simulink model "Exercitiul4_1"  (R2016a)
settings: Solver=VariableStepDiscrete  StartTime=0.0  StopTime=100  RelTol=1e-3
undefined symbols (not defined in the file): exprnd, m
settings Model: Creator=Cristina  LastModifiedBy=Cristina

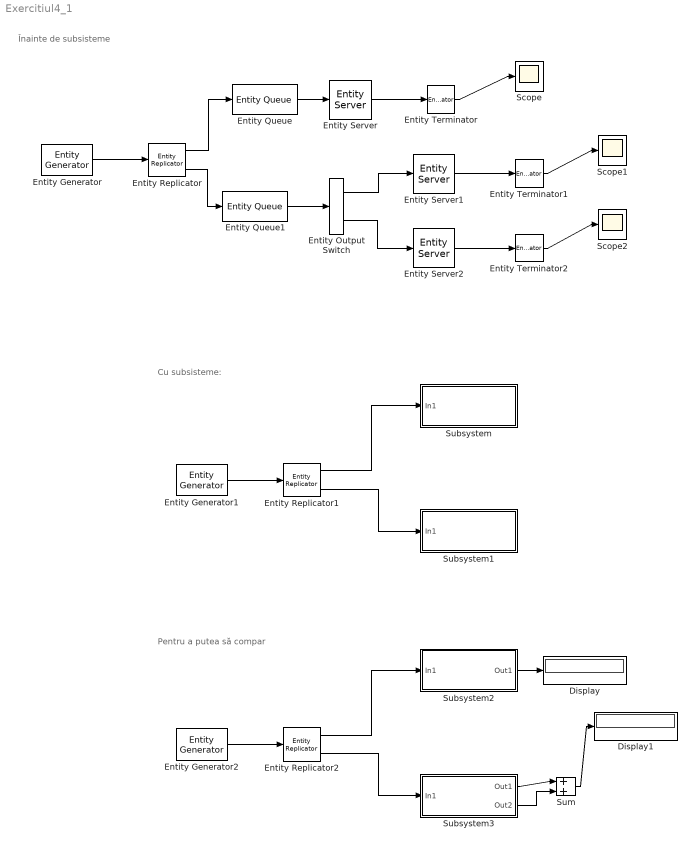
== system Exercitiul4_1 ==
  note: Cu subsisteme:
  note: Înainte de subsisteme
  note: Pentru a putea să compar
  Display : Display
  Display1 : Display
  Entity Output Switch : EntityOutputSwitch  InputPortMessageModes=m  OutputPortMessageModes=m,m  SwitchAttributeName=Attribute1
  Entity Generator : EntityGenerator  OutputPortMessageModes=m  TimeSource=MATLAB action  IntergenerationTimeAction=dt = exprnd(0.5);  AttributeName=ServiceTime  AttributeInitialValue=exprnd(1)  EntityType=Structured  EntityTypeName=Entity
  Entity Generator1 : EntityGenerator  OutputPortMessageModes=m  TimeSource=MATLAB action  IntergenerationTimeAction=dt = exprnd(0.5);  AttributeName=ServiceTime  AttributeInitialValue=exprnd(1)  EntityType=Structured  EntityTypeName=Entity
  Entity Generator2 : EntityGenerator  OutputPortMessageModes=m  TimeSource=MATLAB action  IntergenerationTimeAction=dt = exprnd(0.5);  AttributeName=ServiceTime  AttributeInitialValue=exprnd(1)  EntityType=Structured  EntityTypeName=Entity
  Entity Queue : EntityQueue  InputPortMessageModes=m  OutputPortMessageModes=m
      settings: OutputPortMap=o5
  Entity Queue1 : EntityQueue  InputPortMessageModes=m  OutputPortMessageModes=m
      settings: OutputPortMap=o5
  Entity Replicator : EntityReplicator  InputPortMessageModes=m  OutputPortMessageModes=m,m
  Entity Replicator1 : EntityReplicator  InputPortMessageModes=m  OutputPortMessageModes=m,m
  Entity Replicator2 : EntityReplicator  InputPortMessageModes=m  OutputPortMessageModes=m,m
  Entity Server : EntityServer  InputPortMessageModes=m  OutputPortMessageModes=m  Capacity=2  ServiceTimeSource=Attribute
  Entity Server1 : EntityServer  InputPortMessageModes=m  OutputPortMessageModes=m  Capacity=1  ServiceTimeSource=Attribute
  Entity Server2 : EntityServer  InputPortMessageModes=m  OutputPortMessageModes=m  Capacity=1  ServiceTimeSource=Attribute
  Entity Terminator : EntityTerminator  InputPortMessageModes=m  NumberEntitiesArrived=on
      settings: OutputPortMap=o0
  Entity Terminator1 : EntityTerminator  InputPortMessageModes=m  NumberEntitiesArrived=on
      settings: OutputPortMap=o0
  Entity Terminator2 : EntityTerminator  InputPortMessageModes=m  NumberEntitiesArrived=on
      settings: OutputPortMap=o0
  Scope : Scope
  Scope1 : Scope
  Scope2 : Scope
  Subsystem : Subsystem
  Subsystem1 : Subsystem
  Subsystem2 : Subsystem
  Subsystem3 : Subsystem
  Sum : Sum  Inputs=|++
  wires:
  Entity Replicator/1 -> Entity Queue/1
  Entity Generator/1 -> Entity Replicator/1
  Entity Replicator/2 -> Entity Queue1/1
  Entity Queue/1 -> Entity Server/1
  Entity Queue1/1 -> Entity Output Switch/1
  Entity Output Switch/1 -> Entity Server1/1
  Entity Output Switch/2 -> Entity Server2/1
  Entity Server/1 -> Entity Terminator/1
  Entity Server1/1 -> Entity Terminator1/1
  Entity Server2/1 -> Entity Terminator2/1
  Entity Terminator/1 -> Scope/1
  Entity Terminator1/1 -> Scope1/1
  Entity Terminator2/1 -> Scope2/1
  Entity Generator1/1 -> Entity Replicator1/1
  Entity Replicator1/2 -> Subsystem1/1(In1)
  Entity Replicator1/1 -> Subsystem/1(In1)
  Entity Generator2/1 -> Entity Replicator2/1
  Entity Replicator2/2 -> Subsystem3/1(In1)
  Entity Replicator2/1 -> Subsystem2/1(In1)
  Subsystem2/1(Out1) -> Display/1
  Subsystem3/1(Out1) -> Sum/1
  Subsystem3/2(Out2) -> Sum/2
  Sum/1 -> Display1/1

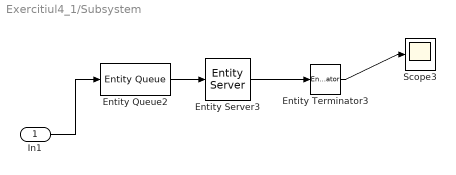
== system Exercitiul4_1/Subsystem ==
  In1 : Inport
  Entity Queue2 : EntityQueue  InputPortMessageModes=m  OutputPortMessageModes=m
      settings: OutputPortMap=o5
  Entity Server3 : EntityServer  InputPortMessageModes=m  OutputPortMessageModes=m  Capacity=2  ServiceTimeSource=Attribute
  Entity Terminator3 : EntityTerminator  InputPortMessageModes=m  NumberEntitiesArrived=on
      settings: OutputPortMap=o0
  Scope3 : Scope
  wires:
  In1/1 -> Entity Queue2/1
  Entity Queue2/1 -> Entity Server3/1
  Entity Server3/1 -> Entity Terminator3/1
  Entity Terminator3/1 -> Scope3/1

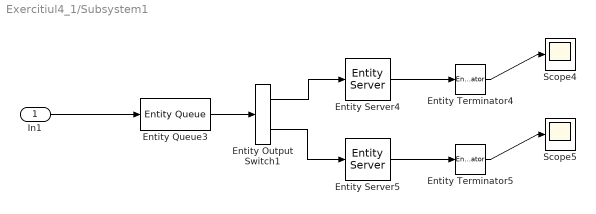
== system Exercitiul4_1/Subsystem1 ==
  In1 : Inport
  Entity Output Switch1 : EntityOutputSwitch  InputPortMessageModes=m  OutputPortMessageModes=m,m  SwitchAttributeName=Attribute1
  Entity Queue3 : EntityQueue  InputPortMessageModes=m  OutputPortMessageModes=m
      settings: OutputPortMap=o5
  Entity Server4 : EntityServer  InputPortMessageModes=m  OutputPortMessageModes=m  Capacity=1  ServiceTimeSource=Attribute
  Entity Server5 : EntityServer  InputPortMessageModes=m  OutputPortMessageModes=m  Capacity=1  ServiceTimeSource=Attribute
  Entity Terminator4 : EntityTerminator  InputPortMessageModes=m  NumberEntitiesArrived=on
      settings: OutputPortMap=o0
  Entity Terminator5 : EntityTerminator  InputPortMessageModes=m  NumberEntitiesArrived=on
      settings: OutputPortMap=o0
  Scope4 : Scope
  Scope5 : Scope
  wires:
  Entity Queue3/1 -> Entity Output Switch1/1
  Entity Output Switch1/1 -> Entity Server4/1
  Entity Output Switch1/2 -> Entity Server5/1
  Entity Server4/1 -> Entity Terminator4/1
  Entity Server5/1 -> Entity Terminator5/1
  Entity Terminator4/1 -> Scope4/1
  Entity Terminator5/1 -> Scope5/1
  In1/1 -> Entity Queue3/1

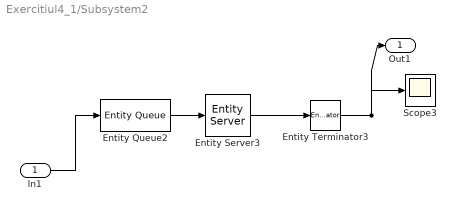
== system Exercitiul4_1/Subsystem2 ==
  In1 : Inport
  Entity Queue2 : EntityQueue  InputPortMessageModes=m  OutputPortMessageModes=m
      settings: OutputPortMap=o5
  Entity Server3 : EntityServer  InputPortMessageModes=m  OutputPortMessageModes=m  Capacity=2  ServiceTimeSource=Attribute
  Entity Terminator3 : EntityTerminator  InputPortMessageModes=m  NumberEntitiesArrived=on
      settings: OutputPortMap=o0
  Scope3 : Scope
  Out1 : Outport
  wires:
  Entity Terminator3/1 -> Out1/1, Scope3/1
  Entity Server3/1 -> Entity Terminator3/1
  Entity Queue2/1 -> Entity Server3/1
  In1/1 -> Entity Queue2/1

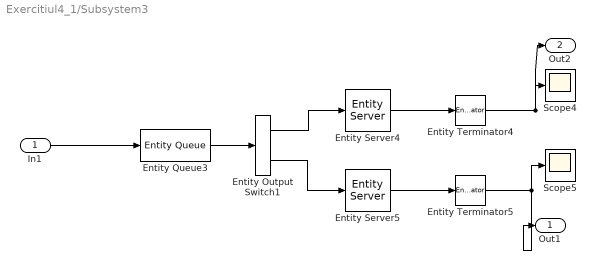
== system Exercitiul4_1/Subsystem3 ==
  In1 : Inport
  Entity Output Switch1 : EntityOutputSwitch  InputPortMessageModes=m  OutputPortMessageModes=m,m  SwitchAttributeName=Attribute1
  Entity Queue3 : EntityQueue  InputPortMessageModes=m  OutputPortMessageModes=m
      settings: OutputPortMap=o5
  Entity Server4 : EntityServer  InputPortMessageModes=m  OutputPortMessageModes=m  Capacity=1  ServiceTimeSource=Attribute
  Entity Server5 : EntityServer  InputPortMessageModes=m  OutputPortMessageModes=m  Capacity=1  ServiceTimeSource=Attribute
  Entity Terminator4 : EntityTerminator  InputPortMessageModes=m  NumberEntitiesArrived=on
      settings: OutputPortMap=o0
  Entity Terminator5 : EntityTerminator  InputPortMessageModes=m  NumberEntitiesArrived=on
      settings: OutputPortMap=o0
  Scope4 : Scope
  Scope5 : Scope
  Out1 : Outport
  Out2 : Outport  Port=2
  wires:
  In1/1 -> Entity Queue3/1
  Entity Terminator5/1 -> Out1/1, Scope5/1
  Entity Server5/1 -> Entity Terminator5/1
  Entity Server4/1 -> Entity Terminator4/1
  Entity Output Switch1/2 -> Entity Server5/1
  Entity Output Switch1/1 -> Entity Server4/1
  Entity Queue3/1 -> Entity Output Switch1/1
  Entity Terminator4/1 -> Out2/1, Scope4/1
